simulink model "gm_model_eq_wfa_interface_old"  (R2020b)
settings: Solver=FixedStepAuto  StartTime=0.0  StopTime=2e-3  RelTol=1e-3  EnableMultiTasking=on
values from neighbouring files (symbols this model uses):
  Ts = 1e-3    (= 0.001)    [compute_constants.m]    (also in signat_to_test_generate.m)
undefined symbols (not defined in the file or in its folder): ip
libraries: axi_iio_lib x2
settings Model: Creator=pablo  LastModifiedBy=pablo
settings SolverCC: ConcurrentTasks=on  PositivePriorityOrder=on
settings OptimizationCC: EnhancedBackFolding=on  PassReuseOutputArgsAs=Individual arguments  ZeroExternalMemoryAtStartup=off  ZeroInternalMemoryAtStartup=off  MaxStackSize=64  OptimizeBlockOrder=speed  DifferentSizesBufferReuse=on  OptimizationCustomize=off  EfficientTunableParamExpr=on
settings DebuggingCC: ParameterTunabilityLossMsg=error
settings HardwareCC: ProdBitPerPointer=32  ProdBitPerSizeT=32  ProdBitPerPtrDiffT=32  ProdLargestAtomicInteger=Long  ProdLargestAtomicFloat=Double  ProdWordSize=32  ProdLongLongMode=on  ProdHWDeviceType=ARM Compatible->ARM Cortex  TargetBitPerPointer=64  TargetBitPerSizeT=64  TargetBitPerPtrDiffT=64  TargetLargestAtomicFloat=Float  TargetIntDivRoundTo=Zero  TargetEndianess=LittleEndian  TargetWordSize=64  TargetHWDeviceType=Intel->x86-64 (Windows64)
settings SFSimCC: MATLABDynamicMemAlloc=off
settings RTWCC: Description=Embedded Coder  SystemTargetFile=ert.tlc  HardwareBoard=Xilinx Zynq-7000 based board  TLCOptions="-aInlineSetEventsForThisBaseRateFcn=TLC_FALSE -aSuppressMultiTaskScheduler=TLC_FALSE  -aRateBasedStepFcn=0"  TemplateMakefile=ert_default_tmf  Toolchain=Linaro AArch32 Linux v6.3.1
settings CodeAppCC: ForceParamTrailComments=on  IgnoreCustomStorageClasses=off  OperatorAnnotations=on  SimulinkDataObjDesc=on  SFDataObjDesc=on  InsertBlockDesc=on

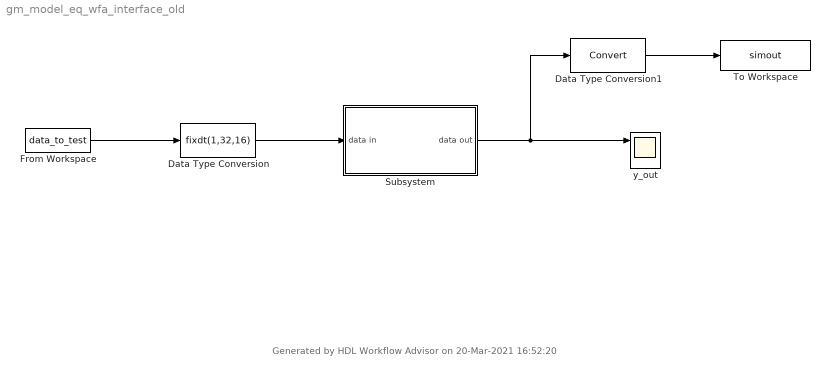
== system gm_model_eq_wfa_interface_old ==
  note: Generated by HDL Workflow Advisor on 20-Mar-2021 16:52:20
  Data Type Conversion : DataTypeConversion  OutDataTypeStr=fixdt(1,32,16)
  Data Type Conversion1 : DataTypeConversion
  From Workspace : FromWorkspace  VariableName=data_to_test  SampleTime=Ts  Interpolate=off  OutputAfterFinalValue=Cyclic repetition
  Subsystem : Subsystem
  To Workspace : ToWorkspace  VariableName=simout  SampleTime=Ts
  y_out : Scope  NumInputPorts=2
  wires:
  From Workspace/1 -> Data Type Conversion/1
  Subsystem/1(data out) -> Data Type Conversion1/1, y_out/1
  Data Type Conversion/1 -> Subsystem/1(data in)
  Data Type Conversion1/1 -> To Workspace/1

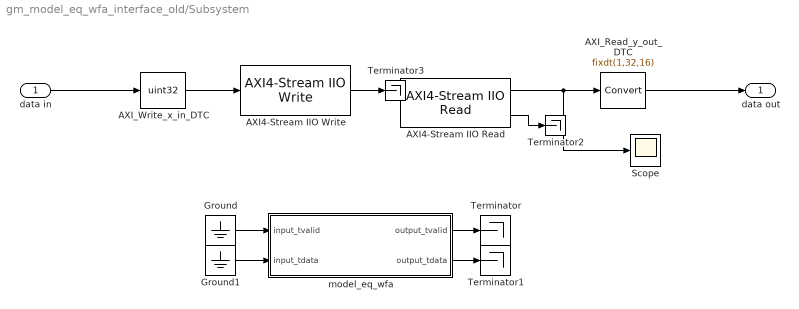
== system gm_model_eq_wfa_interface_old/Subsystem ==
  data in : Inport
  AXI4-Stream IIO Read : axi_iio_lib/AXI4-Stream IIO Read  devName=mwipcore0:s2mm0  SamplesPerFrame=32  dataTypeStr=uint32  tLastMode=auto  resetTlastMode=prebuffer  SampleTime=Ts  DataTimeout=10  uri=ip:10.0.0.200  enIO=off
      settings: SourceProductBaseCode=HDL_ALTERA_SOC,INTEL_FPGA_SOC,XILINX_FPGA_SOC,INTEL_BLOCKSET,USRPEMBED,XILINX_BLOCKSET,HCZYNQ7000,ECZYNQ7000,XILINXZYNQ,VP_VISION_ZYNQ
  AXI4-Stream IIO Write : axi_iio_lib/AXI4-Stream IIO Write  Priority=1  devName=mwipcore0:mm2s0  DataTimeout=0  uri=ip:10.0.0.200  enIO=off
      settings: SourceProductBaseCode=HDL_ALTERA_SOC,INTEL_FPGA_SOC,XILINX_FPGA_SOC,INTEL_BLOCKSET,USRPEMBED,XILINX_BLOCKSET,HCZYNQ7000,ECZYNQ7000,XILINXZYNQ,VP_VISION_ZYNQ
  AXI_Read_y_out_DTC : DataTypeConversion  OutDataTypeStr=fixdt(1,32,16)  ConvertRealWorld=Stored Integer (SI)
  AXI_Write_x_in_DTC : DataTypeConversion  OutDataTypeStr=uint32  ConvertRealWorld=Stored Integer (SI)
  Ground : Ground
  Ground1 : Ground
  Scope : Scope
  Terminator{,1..3} (4 alike) : Terminator
  model_eq_wfa : Subsystem  TreatAsAtomicUnit=on  mask(AXI4-Lite/AXI4 Interface){}
      mask help:
      | This is an automatically generated subsystem block.
      | This contains the AXI interface blocks that communicate with the axis_goertzel_ip IPCore generated from model_eq_wfa subsystem.
      mask Display: disp(sprintf('Xilinx Zynq \nAXI Interface'));
  data out : Outport
  wires:
  AXI4-Stream IIO Read/2 -> Terminator2/1
  AXI_Read_y_out_DTC/1 -> data out/1
  Ground/1 -> model_eq_wfa/1(input_tvalid)
  model_eq_wfa/1(output_tvalid) -> Terminator/1
  AXI_Write_x_in_DTC/1 -> AXI4-Stream IIO Write/1
  data in/1 -> AXI_Write_x_in_DTC/1
  model_eq_wfa/2(output_tdata) -> Terminator1/1
  AXI4-Stream IIO Write/1 -> Terminator3/1
  AXI4-Stream IIO Read/1 -> Scope/1, AXI_Read_y_out_DTC/1
  Ground1/1 -> model_eq_wfa/2(input_tdata)

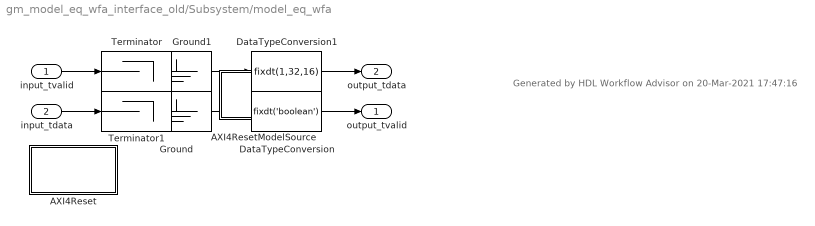
== system gm_model_eq_wfa_interface_old/Subsystem/model_eq_wfa ==
  note: Generated by HDL Workflow Advisor on 20-Mar-2021 17:47:16
  input_tvalid : Inport
  input_tdata : Inport  Port=2
  AXI4Reset : Subsystem  mask(System Start){ShowInLibBrowser=0}
      mask prompts: ShowInLibBrowser "Simulink:masks:CustCodeMaskParam1_MP"
      settings: CopyFcn=cccopyfcn(gcb)  OpenFcn=ccopenfcn('System Start Function')
      mask Help: eval('feval(''rtwprivate'',''rtwhelpview'',''rtw_sys_start_block'')');
      mask Display: disp('System\nStart');
  AXI4ResetModelSource : Subsystem  mask(Model Source){ShowInLibBrowser=0}
      mask prompts: ShowInLibBrowser "Simulink:masks:CustCodeMaskParam1_MP"
      settings: CopyFcn=cccopyfcn(gcb)  OpenFcn=ccopenfcn('Model Source')
      mask Help: eval('feval(''rtwprivate'',''rtwhelpview'',''rtw_model_source_block'')');
      mask Display: disp('Model\nSource');
  DataTypeConversion : DataTypeConversion  OutDataTypeStr=fixdt('boolean')  ConvertRealWorld=Stored Integer (SI)
  DataTypeConversion1 : DataTypeConversion  OutDataTypeStr=fixdt(1,32,16)  ConvertRealWorld=Stored Integer (SI)
  Ground : Ground
  Ground1 : Ground
  Terminator : Terminator
  Terminator1 : Terminator
  output_tvalid : Outport
  output_tdata : Outport  Port=2
  wires:
  input_tvalid/1 -> Terminator/1
  input_tdata/1 -> Terminator1/1
  DataTypeConversion/1 -> output_tvalid/1
  Ground/1 -> DataTypeConversion/1
  DataTypeConversion1/1 -> output_tdata/1
  Ground1/1 -> DataTypeConversion1/1

== system gm_model_eq_wfa_interface_old/Subsystem/model_eq_wfa/AXI4Reset ==

== system gm_model_eq_wfa_interface_old/Subsystem/model_eq_wfa/AXI4ResetModelSource ==
